simulink model "FTBO_Eq_diff_Vm_oc"  (R2021b)
settings: Solver=VariableStepAuto  StartTime=0.0  StopTime=1.227  RelTol=1e-3
values from neighbouring files (symbols this model uses):
  Eq_diff_coeff_oc = (Bm*Rm+Bc*N^2*Rm+nm*kt*km)/(Rm*(Jm+Jc*N^2))    (= 579.744964975)    [Projet.m]
  Eq_diff_coeff_Vm = (N*nm*kt/(Rm*Jm+Rm*Jc*N^2))    (= 0.166128835867)    [Projet.m]
settings Model: Creator=levm1106  LastModifiedBy=levm1106

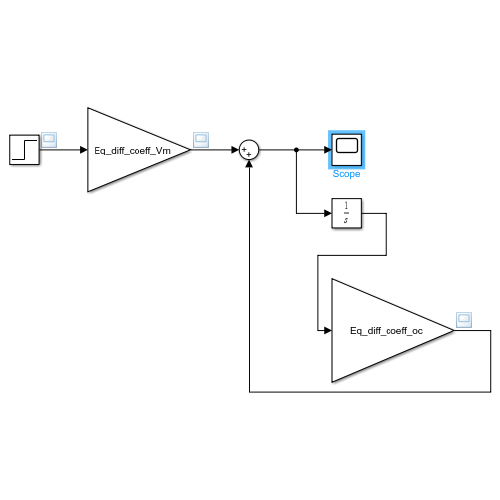
[thumbnail: Simulink's stored preview of the top-level diagram]
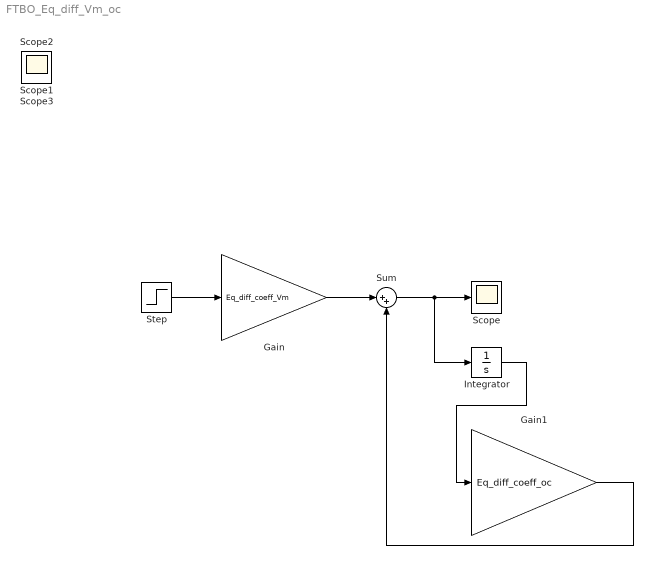
== system FTBO_Eq_diff_Vm_oc ==
  Gain : Gain  Gain=Eq_diff_coeff_Vm
  Gain1 : Gain  Gain=Eq_diff_coeff_oc
  Integrator : Integrator
  Scope{,1..3} (4 alike) : Scope
  Step : Step  Time=0  SampleTime=0
  Sum : Sum  Inputs=|++
  wires:
  Step/1 -> Gain/1
  Gain/1 -> Sum/1
  Sum/1 -> Integrator/1, Scope/1
  Integrator/1 -> Gain1/1
  Gain1/1 -> Sum/2
